simulink model "Boeing787_Yue"  (R2013a)
settings: Solver=ode23tb  SolverMode=SingleTasking  StartTime=0.0  StopTime=346  RelTol=1e-3
InitFcn:
  | load('SampleOutput.mat')
  | 
  | load('SampleFuelBurn.mat')
values from neighbouring files (symbols this model uses):
  FuelBurn = [0 0 0 0 0 0 0 0 0 0 0 0 ... (18249 elements, 1x18249)]    [Benchmark_data1.mat]
undefined symbols (not defined in the file or in its folder): ailerons, AirProp, B_737, elevator, HydProp, landing_gear, rudder, thrust_rev
libraries: PowerFlowLib x118, simulink x20
(part 25 of 26)

== system Boeing787_Yue/Electrical/Generation Unit Sync-Sync2/Generator/Stator Voltage ==
  Id : Inport
  Iq : Inport  Port=2
  Eq1 : Inport  Port=3
  Ed1 : Inport  Port=4
  Phi_1d : Inport  Port=5
  Phi_2q : Inport  Port=6
  w/ws : Inport  Port=7
  Temp : Inport  Port=8
  Gain : Gain  Gain=(Xq2 - Xls)/(Xq1 - Xls)
  Gain1 : Gain  Gain=(Xq1 - Xq2)/(Xq1 - Xls)
  Gain2 : Gain  Gain=(Xq2 - Xd2)
  Gain3 : Gain  Gain=(Xd2 - Xls)/(Xd1 - Xls)
  Gain4 : Gain  Gain=(Xd1 - Xd2)/(Xd1 - Xls)
  Gain5 : Gain  Gain=Rs
  Gain6 : Gain  Gain=Xd2
  Gain7 : Gain  Gain=Rs
  Gain8 : Gain  Gain=Xd2
  Product{,1..3,5} (5 alike) : Product  RndMeth=Zero
  Product4 : Product
  Sum : Sum
  Sum1 : Sum  Inputs=+-+
  Sum2 : Sum  Inputs=--+
  Sum3 : Sum  Inputs=-++
  Ed : Outport
  Eq : Outport  Port=2
  wires:
  Gain7/1 -> Sum2/2
  Product3/1 -> Sum2/1
  Sum2/1 -> Eq/1  "Vq"
  Sum3/1 -> Ed/1  "Vd"
  Product2/1 -> Sum3/3
  Product1/1 -> Sum3/2
  Gain8/1 -> Product3/1
  Gain6/1 -> Product2/2
  Id/1 -> Gain8/1, Gain5/1
  Product/1 -> Sum2/3
  w/ws/1 -> Product2/1, Product3/2, Product/2, Product1/2
  Sum1/1 -> Product1/1
  Sum/1 -> Product/1
  Gain1/1 -> Sum1/2
  Gain/1 -> Sum1/1
  Gain3/1 -> Sum/1
  Gain4/1 -> Sum/2
  Phi_1d/1 -> Gain4/1
  Eq1/1 -> Gain3/1
  Phi_2q/1 -> Gain1/1
  Ed1/1 -> Gain/1
  Gain2/1 -> Sum1/3
  Temp/1 -> Product5/1, Product4/2
  Gain5/1 -> Product4/1
  Product4/1 -> Sum3/1
  Product5/1 -> Gain7/1
  Iq/1 -> Gain2/1, Product5/2, Gain6/1

== system Boeing787_Yue/Electrical/Generation Unit Sync-Sync3/Generator/Dynamics ==
  Id : Inport
  Iq : Inport  Port=2
  Efd : Inport  Port=3
  Temp : Inport  Port=4
  Gain : Gain  Gain=Xd1 - Xls
  Gain1 : Gain  Gain=(Xd1 - Xd2)/(Xd1-Xls)^2
  Gain10 : Gain  Gain=Xq1 - Xls
  Gain11 : Gain  Gain=1/Tqo2
  Gain2 : Gain  Gain=Xd - Xd1
  Gain3 : Gain  Gain=1/Tdo1
  Gain4 : Gain  Gain=Xq1 - Xls
  Gain5 : Gain  Gain=(Xq1 - Xq2)/(Xq1 - Xls)^2
  Gain6 : Gain  Gain=Xq - Xq1
  Gain7 : Gain  Gain=1/Tqo1
  Gain8 : Gain  Gain=Xd1 - Xls
  Gain9 : Gain  Gain=1/Tdo2
  Integrator{,1..3} (4 alike) : Integrator
  Product{1..4} (4 alike) : Product
  Sum : Sum  Inputs=++-
  Sum1 : Sum  Inputs=+-
  Sum2 : Sum  Inputs=--+
  Sum3 : Sum  Inputs=+++
  Sum4 : Sum  Inputs=+-
  Sum5 : Sum  Inputs=-+
  Sum6 : Sum  Inputs=--+
  Sum7 : Sum  Inputs=---
  Eq1 : Outport
  Ed1 : Outport  Port=2
  Phi_1d : Outport  Port=3
  Phi_2q : Outport  Port=4
  wires:
  Efd/1 -> [Efd]
  Iq/1 -> [Iq]
  Id/1 -> [Id]
  Integrator3/1 -> Phi_2q/1, [Phi_2q]
  Sum7/1 -> Gain11/1
  [Ed1] -> Sum7/3
  [Phi_2q] -> Sum7/2
  Gain10/1 -> Sum7/1
  [Iq] -> Gain10/1
  Integrator2/1 -> Phi_1d/1, [Phi_1d]
  Sum6/1 -> Gain9/1
  [Eq1] -> Sum6/3
  [Phi_1d] -> Sum6/2
  Gain8/1 -> Sum6/1
  [Id] -> Gain8/1
  Sum5/1 -> Gain7/1
  Gain6/1 -> Sum5/2
  [Ed1] -> Sum5/1
  Sum4/1 -> Gain6/1
  Gain5/1 -> Sum4/2
  [Iq] -> Sum4/1
  Sum3/1 -> Gain5/1
  [Ed1] -> Sum3/3
  [Phi_2q] -> Sum3/2
  Gain4/1 -> Sum3/1
  [Iq] -> Gain4/1
  Integrator1/1 -> [Ed1], Ed1/1
  Sum2/1 -> Gain3/1
  [Efd] -> Sum2/3
  Gain2/1 -> Sum2/2
  [Eq1] -> Sum2/1
  Sum1/1 -> Gain2/1
  Gain1/1 -> Sum1/2
  [Id] -> Sum1/1
  Sum/1 -> Gain1/1
  [Eq1] -> Sum/3
  [Id] -> Gain/1
  Integrator/1 -> [Eq1], Eq1/1
  Gain/1 -> Sum/1
  [Phi_1d] -> Sum/2
  Temp/1 -> [R_temp_delta]
  [R_temp_delta] -> Product3/1
  Gain9/1 -> Product3/2
  Product3/1 -> Integrator2/1
  [R_temp_delta] -> Product1/1
  Gain11/1 -> Product1/2
  Product1/1 -> Integrator3/1
  [R_temp_delta] -> Product2/1
  Gain3/1 -> Product2/2
  Product2/1 -> Integrator/1
  [R_temp_delta] -> Product4/1
  Gain7/1 -> Product4/2
  Product4/1 -> Integrator1/1

== system Boeing787_Yue/Electrical/Generation Unit Sync-Sync3/Generator/Electromagnetic Torque Output Power ==
  note: Torque from Damper Windings
  note: Torque from Field Winding
  Id : Inport
  Iq : Inport  Port=2
  Eq1 : Inport  Port=3
  Ed1 : Inport  Port=4
  Phi_1d : Inport  Port=5
  Phi_2q : Inport  Port=6
  Gain : Gain  Gain=(Xd2 - Xls)/(Xd1 - Xls)
  Gain1 : Gain  Gain=(Xq2 - Xls)/(Xq1 - Xls)
  Gain2 : Gain  Gain=(Xd1 - Xd2)/(Xd1-Xls)
  Gain3 : Gain  Gain=(Xq1 - Xq2)/(Xq1-Xls)
  Gain4 : Gain  Gain=(Xq2 - Xd2)
  Product{,1..4} (5 alike) : Product  RndMeth=Zero
  Sum : Sum
  Sum1 : Sum  Inputs=+-+
  Sum2 : Sum
  TE : Outport
  wires:
  Sum2/1 -> TE/1
  Sum1/1 -> Sum2/2
  Sum/1 -> Sum2/1
  Gain1/1 -> Sum/2
  Gain/1 -> Sum/1
  Gain4/1 -> Sum1/3
  Gain2/1 -> Sum1/1
  Gain3/1 -> Sum1/2
  Product4/1 -> Gain4/1
  [Iq] -> Product4/2
  [Id] -> Product4/1
  Product3/1 -> Gain3/1
  [Phi_2q] -> Product3/2
  [Id] -> Product3/1
  Product2/1 -> Gain2/1
  [Phi_1d] -> Product2/2
  [Iq] -> Product2/1
  Product1/1 -> Gain1/1
  [Id] -> Product1/2
  [Ed1] -> Product1/1
  Product/1 -> Gain/1
  [Iq] -> Product/2
  [Eq1] -> Product/1
  Iq/1 -> [Iq]
  Phi_2q/1 -> [Phi_2q]
  Phi_1d/1 -> [Phi_1d]
  Ed1/1 -> [Ed1]
  Eq1/1 -> [Eq1]
  Id/1 -> [Id]

== system Boeing787_Yue/Electrical/Generation Unit Sync-Sync3/Generator/Generator Power Loss ==
  Ed : Inport
  Eq : Inport  Port=2
  Id : Inport  Port=3
  Iq : Inport  Port=4
  Te : Inport  Port=5
  w/ws : Inport  Port=6
  Bus Creator : BusCreator  Inputs=6
  Gain1 : Gain  Gain=SB
  Gain2 : Gain  Gain=SB
  Gain3 : Gain  Gain=SB
  Product : Product  RndMeth=Zero
  Product1 : Product  RndMeth=Zero
  Product2 : Product  RndMeth=Zero
  Sum1 : Sum  Inputs=-+
  Sum2 : Sum
  PE : Outport
  PM : Outport  Port=2
  PLOSS : Outport  Port=3
  m : Outport  Port=4
  wires:
  Gain3/1 -> PM/1
  Gain1/1 -> PE/1
  Gain2/1 -> PLOSS/1
  Bus Creator/1 -> m/1
  [nu] -> Bus Creator/6  "nu"
  [Te] -> Bus Creator/5  "Te"
  [Iq] -> Bus Creator/4  "Iq"
  [Eq] -> Bus Creator/3  "Vq"
  [Id] -> Bus Creator/2  "Id"
  [Ed] -> Bus Creator/1  "Vd"
  Sum1/1 -> Gain2/1
  Product2/1 -> Gain3/1, Sum1/2
  Sum2/1 -> Gain1/1, Sum1/1
  Product1/1 -> Sum2/2
  Product/1 -> Sum2/1
  [nu] -> Product2/2
  [Te] -> Product2/1
  [Iq] -> Product1/2
  [Eq] -> Product1/1
  [Id] -> Product/2
  [Ed] -> Product/1
  w/ws/1 -> [nu]
  Te/1 -> [Te]
  Iq/1 -> [Iq]
  Id/1 -> [Id]
  Eq/1 -> [Eq]
  Ed/1 -> [Ed]

== system Boeing787_Yue/Electrical/Generation Unit Sync-Sync3/Generator/Stator Voltage ==
  Id : Inport
  Iq : Inport  Port=2
  Eq1 : Inport  Port=3
  Ed1 : Inport  Port=4
  Phi_1d : Inport  Port=5
  Phi_2q : Inport  Port=6
  w/ws : Inport  Port=7
  Temp : Inport  Port=8
  Gain : Gain  Gain=(Xq2 - Xls)/(Xq1 - Xls)
  Gain1 : Gain  Gain=(Xq1 - Xq2)/(Xq1 - Xls)
  Gain2 : Gain  Gain=(Xq2 - Xd2)
  Gain3 : Gain  Gain=(Xd2 - Xls)/(Xd1 - Xls)
  Gain4 : Gain  Gain=(Xd1 - Xd2)/(Xd1 - Xls)
  Gain5 : Gain  Gain=Rs
  Gain6 : Gain  Gain=Xd2
  Gain7 : Gain  Gain=Rs
  Gain8 : Gain  Gain=Xd2
  Product{,1..3,5} (5 alike) : Product  RndMeth=Zero
  Product4 : Product
  Sum : Sum
  Sum1 : Sum  Inputs=+-+
  Sum2 : Sum  Inputs=--+
  Sum3 : Sum  Inputs=-++
  Ed : Outport
  Eq : Outport  Port=2
  wires:
  Gain7/1 -> Sum2/2
  Product3/1 -> Sum2/1
  Sum2/1 -> Eq/1  "Vq"
  Sum3/1 -> Ed/1  "Vd"
  Product2/1 -> Sum3/3
  Product1/1 -> Sum3/2
  Gain8/1 -> Product3/1
  Gain6/1 -> Product2/2
  Id/1 -> Gain8/1, Gain5/1
  Product/1 -> Sum2/3
  w/ws/1 -> Product2/1, Product3/2, Product/2, Product1/2
  Sum1/1 -> Product1/1
  Sum/1 -> Product/1
  Gain1/1 -> Sum1/2
  Gain/1 -> Sum1/1
  Gain3/1 -> Sum/1
  Gain4/1 -> Sum/2
  Phi_1d/1 -> Gain4/1
  Eq1/1 -> Gain3/1
  Phi_2q/1 -> Gain1/1
  Ed1/1 -> Gain/1
  Gain2/1 -> Sum1/3
  Temp/1 -> Product5/1, Product4/2
  Gain5/1 -> Product4/1
  Product4/1 -> Sum3/1
  Product5/1 -> Gain7/1
  Iq/1 -> Gain2/1, Product5/2, Gain6/1

== system Boeing787_Yue/Electrical/Generation Unit Sync-Sync4/Generator/Dynamics ==
  Id : Inport
  Iq : Inport  Port=2
  Efd : Inport  Port=3
  Temp : Inport  Port=4
  Gain : Gain  Gain=Xd1 - Xls
  Gain1 : Gain  Gain=(Xd1 - Xd2)/(Xd1-Xls)^2
  Gain10 : Gain  Gain=Xq1 - Xls
  Gain11 : Gain  Gain=1/Tqo2
  Gain2 : Gain  Gain=Xd - Xd1
  Gain3 : Gain  Gain=1/Tdo1
  Gain4 : Gain  Gain=Xq1 - Xls
  Gain5 : Gain  Gain=(Xq1 - Xq2)/(Xq1 - Xls)^2
  Gain6 : Gain  Gain=Xq - Xq1
  Gain7 : Gain  Gain=1/Tqo1
  Gain8 : Gain  Gain=Xd1 - Xls
  Gain9 : Gain  Gain=1/Tdo2
  Integrator{,1..3} (4 alike) : Integrator
  Product{1..4} (4 alike) : Product
  Sum : Sum  Inputs=++-
  Sum1 : Sum  Inputs=+-
  Sum2 : Sum  Inputs=--+
  Sum3 : Sum  Inputs=+++
  Sum4 : Sum  Inputs=+-
  Sum5 : Sum  Inputs=-+
  Sum6 : Sum  Inputs=--+
  Sum7 : Sum  Inputs=---
  Eq1 : Outport
  Ed1 : Outport  Port=2
  Phi_1d : Outport  Port=3
  Phi_2q : Outport  Port=4
  wires:
  Efd/1 -> [Efd]
  Iq/1 -> [Iq]
  Id/1 -> [Id]
  Integrator3/1 -> Phi_2q/1, [Phi_2q]
  Sum7/1 -> Gain11/1
  [Ed1] -> Sum7/3
  [Phi_2q] -> Sum7/2
  Gain10/1 -> Sum7/1
  [Iq] -> Gain10/1
  Integrator2/1 -> Phi_1d/1, [Phi_1d]
  Sum6/1 -> Gain9/1
  [Eq1] -> Sum6/3
  [Phi_1d] -> Sum6/2
  Gain8/1 -> Sum6/1
  [Id] -> Gain8/1
  Sum5/1 -> Gain7/1
  Gain6/1 -> Sum5/2
  [Ed1] -> Sum5/1
  Sum4/1 -> Gain6/1
  Gain5/1 -> Sum4/2
  [Iq] -> Sum4/1
  Sum3/1 -> Gain5/1
  [Ed1] -> Sum3/3
  [Phi_2q] -> Sum3/2
  Gain4/1 -> Sum3/1
  [Iq] -> Gain4/1
  Integrator1/1 -> [Ed1], Ed1/1
  Sum2/1 -> Gain3/1
  [Efd] -> Sum2/3
  Gain2/1 -> Sum2/2
  [Eq1] -> Sum2/1
  Sum1/1 -> Gain2/1
  Gain1/1 -> Sum1/2
  [Id] -> Sum1/1
  Sum/1 -> Gain1/1
  [Eq1] -> Sum/3
  [Id] -> Gain/1
  Integrator/1 -> [Eq1], Eq1/1
  Gain/1 -> Sum/1
  [Phi_1d] -> Sum/2
  Temp/1 -> [R_temp_delta]
  [R_temp_delta] -> Product3/1
  Gain9/1 -> Product3/2
  Product3/1 -> Integrator2/1
  [R_temp_delta] -> Product1/1
  Gain11/1 -> Product1/2
  Product1/1 -> Integrator3/1
  [R_temp_delta] -> Product2/1
  Gain3/1 -> Product2/2
  Product2/1 -> Integrator/1
  [R_temp_delta] -> Product4/1
  Gain7/1 -> Product4/2
  Product4/1 -> Integrator1/1

== system Boeing787_Yue/Electrical/Generation Unit Sync-Sync4/Generator/Electromagnetic Torque Output Power ==
  note: Torque from Damper Windings
  note: Torque from Field Winding
  Id : Inport
  Iq : Inport  Port=2
  Eq1 : Inport  Port=3
  Ed1 : Inport  Port=4
  Phi_1d : Inport  Port=5
  Phi_2q : Inport  Port=6
  Gain : Gain  Gain=(Xd2 - Xls)/(Xd1 - Xls)
  Gain1 : Gain  Gain=(Xq2 - Xls)/(Xq1 - Xls)
  Gain2 : Gain  Gain=(Xd1 - Xd2)/(Xd1-Xls)
  Gain3 : Gain  Gain=(Xq1 - Xq2)/(Xq1-Xls)
  Gain4 : Gain  Gain=(Xq2 - Xd2)
  Product{,1..4} (5 alike) : Product  RndMeth=Zero
  Sum : Sum
  Sum1 : Sum  Inputs=+-+
  Sum2 : Sum
  TE : Outport
  wires:
  Sum2/1 -> TE/1
  Sum1/1 -> Sum2/2
  Sum/1 -> Sum2/1
  Gain1/1 -> Sum/2
  Gain/1 -> Sum/1
  Gain4/1 -> Sum1/3
  Gain2/1 -> Sum1/1
  Gain3/1 -> Sum1/2
  Product4/1 -> Gain4/1
  [Iq] -> Product4/2
  [Id] -> Product4/1
  Product3/1 -> Gain3/1
  [Phi_2q] -> Product3/2
  [Id] -> Product3/1
  Product2/1 -> Gain2/1
  [Phi_1d] -> Product2/2
  [Iq] -> Product2/1
  Product1/1 -> Gain1/1
  [Id] -> Product1/2
  [Ed1] -> Product1/1
  Product/1 -> Gain/1
  [Iq] -> Product/2
  [Eq1] -> Product/1
  Iq/1 -> [Iq]
  Phi_2q/1 -> [Phi_2q]
  Phi_1d/1 -> [Phi_1d]
  Ed1/1 -> [Ed1]
  Eq1/1 -> [Eq1]
  Id/1 -> [Id]

== system Boeing787_Yue/Electrical/Generation Unit Sync-Sync4/Generator/Generator Power Loss ==
  Ed : Inport
  Eq : Inport  Port=2
  Id : Inport  Port=3
  Iq : Inport  Port=4
  Te : Inport  Port=5
  w/ws : Inport  Port=6
  Bus Creator : BusCreator  Inputs=6
  Gain1 : Gain  Gain=SB
  Gain2 : Gain  Gain=SB
  Gain3 : Gain  Gain=SB
  Product : Product  RndMeth=Zero
  Product1 : Product  RndMeth=Zero
  Product2 : Product  RndMeth=Zero
  Sum1 : Sum  Inputs=-+
  Sum2 : Sum
  PE : Outport
  PM : Outport  Port=2
  PLOSS : Outport  Port=3
  m : Outport  Port=4
  wires:
  Gain3/1 -> PM/1
  Gain1/1 -> PE/1
  Gain2/1 -> PLOSS/1
  Bus Creator/1 -> m/1
  [nu] -> Bus Creator/6  "nu"
  [Te] -> Bus Creator/5  "Te"
  [Iq] -> Bus Creator/4  "Iq"
  [Eq] -> Bus Creator/3  "Vq"
  [Id] -> Bus Creator/2  "Id"
  [Ed] -> Bus Creator/1  "Vd"
  Sum1/1 -> Gain2/1
  Product2/1 -> Gain3/1, Sum1/2
  Sum2/1 -> Gain1/1, Sum1/1
  Product1/1 -> Sum2/2
  Product/1 -> Sum2/1
  [nu] -> Product2/2
  [Te] -> Product2/1
  [Iq] -> Product1/2
  [Eq] -> Product1/1
  [Id] -> Product/2
  [Ed] -> Product/1
  w/ws/1 -> [nu]
  Te/1 -> [Te]
  Iq/1 -> [Iq]
  Id/1 -> [Id]
  Eq/1 -> [Eq]
  Ed/1 -> [Ed]

== system Boeing787_Yue/Electrical/Generation Unit Sync-Sync4/Generator/Stator Voltage ==
  Id : Inport
  Iq : Inport  Port=2
  Eq1 : Inport  Port=3
  Ed1 : Inport  Port=4
  Phi_1d : Inport  Port=5
  Phi_2q : Inport  Port=6
  w/ws : Inport  Port=7
  Temp : Inport  Port=8
  Gain : Gain  Gain=(Xq2 - Xls)/(Xq1 - Xls)
  Gain1 : Gain  Gain=(Xq1 - Xq2)/(Xq1 - Xls)
  Gain2 : Gain  Gain=(Xq2 - Xd2)
  Gain3 : Gain  Gain=(Xd2 - Xls)/(Xd1 - Xls)
  Gain4 : Gain  Gain=(Xd1 - Xd2)/(Xd1 - Xls)
  Gain5 : Gain  Gain=Rs
  Gain6 : Gain  Gain=Xd2
  Gain7 : Gain  Gain=Rs
  Gain8 : Gain  Gain=Xd2
  Product{,1..3,5} (5 alike) : Product  RndMeth=Zero
  Product4 : Product
  Sum : Sum
  Sum1 : Sum  Inputs=+-+
  Sum2 : Sum  Inputs=--+
  Sum3 : Sum  Inputs=-++
  Ed : Outport
  Eq : Outport  Port=2
  wires:
  Gain7/1 -> Sum2/2
  Product3/1 -> Sum2/1
  Sum2/1 -> Eq/1  "Vq"
  Sum3/1 -> Ed/1  "Vd"
  Product2/1 -> Sum3/3
  Product1/1 -> Sum3/2
  Gain8/1 -> Product3/1
  Gain6/1 -> Product2/2
  Id/1 -> Gain8/1, Gain5/1
  Product/1 -> Sum2/3
  w/ws/1 -> Product2/1, Product3/2, Product/2, Product1/2
  Sum1/1 -> Product1/1
  Sum/1 -> Product/1
  Gain1/1 -> Sum1/2
  Gain/1 -> Sum1/1
  Gain3/1 -> Sum/1
  Gain4/1 -> Sum/2
  Phi_1d/1 -> Gain4/1
  Eq1/1 -> Gain3/1
  Phi_2q/1 -> Gain1/1
  Ed1/1 -> Gain/1
  Gain2/1 -> Sum1/3
  Temp/1 -> Product5/1, Product4/2
  Gain5/1 -> Product4/1
  Product4/1 -> Sum3/1
  Product5/1 -> Gain7/1
  Iq/1 -> Gain2/1, Product5/2, Gain6/1

== system Boeing787_Yue/Electrical/Generation Unit Sync-Sync5/Generator/Dynamics ==
  Id : Inport
  Iq : Inport  Port=2
  Efd : Inport  Port=3
  Temp : Inport  Port=4
  Gain : Gain  Gain=Xd1 - Xls
  Gain1 : Gain  Gain=(Xd1 - Xd2)/(Xd1-Xls)^2
  Gain10 : Gain  Gain=Xq1 - Xls
  Gain11 : Gain  Gain=1/Tqo2
  Gain2 : Gain  Gain=Xd - Xd1
  Gain3 : Gain  Gain=1/Tdo1
  Gain4 : Gain  Gain=Xq1 - Xls
  Gain5 : Gain  Gain=(Xq1 - Xq2)/(Xq1 - Xls)^2
  Gain6 : Gain  Gain=Xq - Xq1
  Gain7 : Gain  Gain=1/Tqo1
  Gain8 : Gain  Gain=Xd1 - Xls
  Gain9 : Gain  Gain=1/Tdo2
  Integrator{,1..3} (4 alike) : Integrator
  Product{1..4} (4 alike) : Product
  Sum : Sum  Inputs=++-
  Sum1 : Sum  Inputs=+-
  Sum2 : Sum  Inputs=--+
  Sum3 : Sum  Inputs=+++
  Sum4 : Sum  Inputs=+-
  Sum5 : Sum  Inputs=-+
  Sum6 : Sum  Inputs=--+
  Sum7 : Sum  Inputs=---
  Eq1 : Outport
  Ed1 : Outport  Port=2
  Phi_1d : Outport  Port=3
  Phi_2q : Outport  Port=4
  wires:
  Efd/1 -> [Efd]
  Iq/1 -> [Iq]
  Id/1 -> [Id]
  Integrator3/1 -> Phi_2q/1, [Phi_2q]
  Sum7/1 -> Gain11/1
  [Ed1] -> Sum7/3
  [Phi_2q] -> Sum7/2
  Gain10/1 -> Sum7/1
  [Iq] -> Gain10/1
  Integrator2/1 -> Phi_1d/1, [Phi_1d]
  Sum6/1 -> Gain9/1
  [Eq1] -> Sum6/3
  [Phi_1d] -> Sum6/2
  Gain8/1 -> Sum6/1
  [Id] -> Gain8/1
  Sum5/1 -> Gain7/1
  Gain6/1 -> Sum5/2
  [Ed1] -> Sum5/1
  Sum4/1 -> Gain6/1
  Gain5/1 -> Sum4/2
  [Iq] -> Sum4/1
  Sum3/1 -> Gain5/1
  [Ed1] -> Sum3/3
  [Phi_2q] -> Sum3/2
  Gain4/1 -> Sum3/1
  [Iq] -> Gain4/1
  Integrator1/1 -> [Ed1], Ed1/1
  Sum2/1 -> Gain3/1
  [Efd] -> Sum2/3
  Gain2/1 -> Sum2/2
  [Eq1] -> Sum2/1
  Sum1/1 -> Gain2/1
  Gain1/1 -> Sum1/2
  [Id] -> Sum1/1
  Sum/1 -> Gain1/1
  [Eq1] -> Sum/3
  [Id] -> Gain/1
  Integrator/1 -> [Eq1], Eq1/1
  Gain/1 -> Sum/1
  [Phi_1d] -> Sum/2
  Temp/1 -> [R_temp_delta]
  [R_temp_delta] -> Product3/1
  Gain9/1 -> Product3/2
  Product3/1 -> Integrator2/1
  [R_temp_delta] -> Product1/1
  Gain11/1 -> Product1/2
  Product1/1 -> Integrator3/1
  [R_temp_delta] -> Product2/1
  Gain3/1 -> Product2/2
  Product2/1 -> Integrator/1
  [R_temp_delta] -> Product4/1
  Gain7/1 -> Product4/2
  Product4/1 -> Integrator1/1

== system Boeing787_Yue/Electrical/Generation Unit Sync-Sync5/Generator/Electromagnetic Torque Output Power ==
  note: Torque from Damper Windings
  note: Torque from Field Winding
  Id : Inport
  Iq : Inport  Port=2
  Eq1 : Inport  Port=3
  Ed1 : Inport  Port=4
  Phi_1d : Inport  Port=5
  Phi_2q : Inport  Port=6
  Gain : Gain  Gain=(Xd2 - Xls)/(Xd1 - Xls)
  Gain1 : Gain  Gain=(Xq2 - Xls)/(Xq1 - Xls)
  Gain2 : Gain  Gain=(Xd1 - Xd2)/(Xd1-Xls)
  Gain3 : Gain  Gain=(Xq1 - Xq2)/(Xq1-Xls)
  Gain4 : Gain  Gain=(Xq2 - Xd2)
  Product{,1..4} (5 alike) : Product  RndMeth=Zero
  Sum : Sum
  Sum1 : Sum  Inputs=+-+
  Sum2 : Sum
  TE : Outport
  wires:
  Sum2/1 -> TE/1
  Sum1/1 -> Sum2/2
  Sum/1 -> Sum2/1
  Gain1/1 -> Sum/2
  Gain/1 -> Sum/1
  Gain4/1 -> Sum1/3
  Gain2/1 -> Sum1/1
  Gain3/1 -> Sum1/2
  Product4/1 -> Gain4/1
  [Iq] -> Product4/2
  [Id] -> Product4/1
  Product3/1 -> Gain3/1
  [Phi_2q] -> Product3/2
  [Id] -> Product3/1
  Product2/1 -> Gain2/1
  [Phi_1d] -> Product2/2
  [Iq] -> Product2/1
  Product1/1 -> Gain1/1
  [Id] -> Product1/2
  [Ed1] -> Product1/1
  Product/1 -> Gain/1
  [Iq] -> Product/2
  [Eq1] -> Product/1
  Iq/1 -> [Iq]
  Phi_2q/1 -> [Phi_2q]
  Phi_1d/1 -> [Phi_1d]
  Ed1/1 -> [Ed1]
  Eq1/1 -> [Eq1]
  Id/1 -> [Id]

== system Boeing787_Yue/Electrical/Generation Unit Sync-Sync5/Generator/Generator Power Loss ==
  Ed : Inport
  Eq : Inport  Port=2
  Id : Inport  Port=3
  Iq : Inport  Port=4
  Te : Inport  Port=5
  w/ws : Inport  Port=6
  Bus Creator : BusCreator  Inputs=6
  Gain1 : Gain  Gain=SB
  Gain2 : Gain  Gain=SB
  Gain3 : Gain  Gain=SB
  Product : Product  RndMeth=Zero
  Product1 : Product  RndMeth=Zero
  Product2 : Product  RndMeth=Zero
  Sum1 : Sum  Inputs=-+
  Sum2 : Sum
  PE : Outport
  PM : Outport  Port=2
  PLOSS : Outport  Port=3
  m : Outport  Port=4
  wires:
  Gain3/1 -> PM/1
  Gain1/1 -> PE/1
  Gain2/1 -> PLOSS/1
  Bus Creator/1 -> m/1
  [nu] -> Bus Creator/6  "nu"
  [Te] -> Bus Creator/5  "Te"
  [Iq] -> Bus Creator/4  "Iq"
  [Eq] -> Bus Creator/3  "Vq"
  [Id] -> Bus Creator/2  "Id"
  [Ed] -> Bus Creator/1  "Vd"
  Sum1/1 -> Gain2/1
  Product2/1 -> Gain3/1, Sum1/2
  Sum2/1 -> Gain1/1, Sum1/1
  Product1/1 -> Sum2/2
  Product/1 -> Sum2/1
  [nu] -> Product2/2
  [Te] -> Product2/1
  [Iq] -> Product1/2
  [Eq] -> Product1/1
  [Id] -> Product/2
  [Ed] -> Product/1
  w/ws/1 -> [nu]
  Te/1 -> [Te]
  Iq/1 -> [Iq]
  Id/1 -> [Id]
  Eq/1 -> [Eq]
  Ed/1 -> [Ed]

== system Boeing787_Yue/Electrical/Generation Unit Sync-Sync5/Generator/Stator Voltage ==
  Id : Inport
  Iq : Inport  Port=2
  Eq1 : Inport  Port=3
  Ed1 : Inport  Port=4
  Phi_1d : Inport  Port=5
  Phi_2q : Inport  Port=6
  w/ws : Inport  Port=7
  Temp : Inport  Port=8
  Gain : Gain  Gain=(Xq2 - Xls)/(Xq1 - Xls)
  Gain1 : Gain  Gain=(Xq1 - Xq2)/(Xq1 - Xls)
  Gain2 : Gain  Gain=(Xq2 - Xd2)
  Gain3 : Gain  Gain=(Xd2 - Xls)/(Xd1 - Xls)
  Gain4 : Gain  Gain=(Xd1 - Xd2)/(Xd1 - Xls)
  Gain5 : Gain  Gain=Rs
  Gain6 : Gain  Gain=Xd2
  Gain7 : Gain  Gain=Rs
  Gain8 : Gain  Gain=Xd2
  Product{,1..3,5} (5 alike) : Product  RndMeth=Zero
  Product4 : Product
  Sum : Sum
  Sum1 : Sum  Inputs=+-+
  Sum2 : Sum  Inputs=--+
  Sum3 : Sum  Inputs=-++
  Ed : Outport
  Eq : Outport  Port=2
  wires:
  Gain7/1 -> Sum2/2
  Product3/1 -> Sum2/1
  Sum2/1 -> Eq/1  "Vq"
  Sum3/1 -> Ed/1  "Vd"
  Product2/1 -> Sum3/3
  Product1/1 -> Sum3/2
  Gain8/1 -> Product3/1
  Gain6/1 -> Product2/2
  Id/1 -> Gain8/1, Gain5/1
  Product/1 -> Sum2/3
  w/ws/1 -> Product2/1, Product3/2, Product/2, Product1/2
  Sum1/1 -> Product1/1
  Sum/1 -> Product/1
  Gain1/1 -> Sum1/2
  Gain/1 -> Sum1/1
  Gain3/1 -> Sum/1
  Gain4/1 -> Sum/2
  Phi_1d/1 -> Gain4/1
  Eq1/1 -> Gain3/1
  Phi_2q/1 -> Gain1/1
  Ed1/1 -> Gain/1
  Gain2/1 -> Sum1/3
  Temp/1 -> Product5/1, Product4/2
  Gain5/1 -> Product4/1
  Product4/1 -> Sum3/1
  Product5/1 -> Gain7/1
  Iq/1 -> Gain2/1, Product5/2, Gain6/1

== system Boeing787_Yue/Electrical/Generation Unit Sync-Sync6/Generator/Dynamics ==
  Id : Inport
  Iq : Inport  Port=2
  Efd : Inport  Port=3
  Temp : Inport  Port=4
  Gain : Gain  Gain=Xd1 - Xls
  Gain1 : Gain  Gain=(Xd1 - Xd2)/(Xd1-Xls)^2
  Gain10 : Gain  Gain=Xq1 - Xls
  Gain11 : Gain  Gain=1/Tqo2
  Gain2 : Gain  Gain=Xd - Xd1
  Gain3 : Gain  Gain=1/Tdo1
  Gain4 : Gain  Gain=Xq1 - Xls
  Gain5 : Gain  Gain=(Xq1 - Xq2)/(Xq1 - Xls)^2
  Gain6 : Gain  Gain=Xq - Xq1
  Gain7 : Gain  Gain=1/Tqo1
  Gain8 : Gain  Gain=Xd1 - Xls
  Gain9 : Gain  Gain=1/Tdo2
  Integrator{,1..3} (4 alike) : Integrator
  Product{1..4} (4 alike) : Product
  Sum : Sum  Inputs=++-
  Sum1 : Sum  Inputs=+-
  Sum2 : Sum  Inputs=--+
  Sum3 : Sum  Inputs=+++
  Sum4 : Sum  Inputs=+-
  Sum5 : Sum  Inputs=-+
  Sum6 : Sum  Inputs=--+
  Sum7 : Sum  Inputs=---
  Eq1 : Outport
  Ed1 : Outport  Port=2
  Phi_1d : Outport  Port=3
  Phi_2q : Outport  Port=4
  wires:
  Product4/1 -> Integrator1/1
  Gain7/1 -> Product4/2
  [R_temp_delta] -> Product4/1
  Product2/1 -> Integrator/1
  Gain3/1 -> Product2/2
  [R_temp_delta] -> Product2/1
  Product1/1 -> Integrator3/1
  Gain11/1 -> Product1/2
  [R_temp_delta] -> Product1/1
  Product3/1 -> Integrator2/1
  Gain9/1 -> Product3/2
  [R_temp_delta] -> Product3/1
  Temp/1 -> [R_temp_delta]
  [Phi_1d] -> Sum/2
  Gain/1 -> Sum/1
  Integrator/1 -> Eq1/1, [Eq1]
  [Id] -> Gain/1
  [Eq1] -> Sum/3
  Sum/1 -> Gain1/1
  [Id] -> Sum1/1
  Gain1/1 -> Sum1/2
  Sum1/1 -> Gain2/1
  [Eq1] -> Sum2/1
  Gain2/1 -> Sum2/2
  [Efd] -> Sum2/3
  Sum2/1 -> Gain3/1
  Integrator1/1 -> Ed1/1, [Ed1]
  [Iq] -> Gain4/1
  Gain4/1 -> Sum3/1
  [Phi_2q] -> Sum3/2
  [Ed1] -> Sum3/3
  Sum3/1 -> Gain5/1
  [Iq] -> Sum4/1
  Gain5/1 -> Sum4/2
  Sum4/1 -> Gain6/1
  [Ed1] -> Sum5/1
  Gain6/1 -> Sum5/2
  Sum5/1 -> Gain7/1
  [Id] -> Gain8/1
  Gain8/1 -> Sum6/1
  [Phi_1d] -> Sum6/2
  [Eq1] -> Sum6/3
  Sum6/1 -> Gain9/1
  Integrator2/1 -> [Phi_1d], Phi_1d/1
  [Iq] -> Gain10/1
  Gain10/1 -> Sum7/1
  [Phi_2q] -> Sum7/2
  [Ed1] -> Sum7/3
  Sum7/1 -> Gain11/1
  Integrator3/1 -> [Phi_2q], Phi_2q/1
  Id/1 -> [Id]
  Iq/1 -> [Iq]
  Efd/1 -> [Efd]

== system Boeing787_Yue/Electrical/Generation Unit Sync-Sync6/Generator/Electromagnetic Torque Output Power ==
  note: Torque from Field Winding
  note: Torque from Damper Windings
  Id : Inport
  Iq : Inport  Port=2
  Eq1 : Inport  Port=3
  Ed1 : Inport  Port=4
  Phi_1d : Inport  Port=5
  Phi_2q : Inport  Port=6
  Gain : Gain  Gain=(Xd2 - Xls)/(Xd1 - Xls)
  Gain1 : Gain  Gain=(Xq2 - Xls)/(Xq1 - Xls)
  Gain2 : Gain  Gain=(Xd1 - Xd2)/(Xd1-Xls)
  Gain3 : Gain  Gain=(Xq1 - Xq2)/(Xq1-Xls)
  Gain4 : Gain  Gain=(Xq2 - Xd2)
  Product{,1..4} (5 alike) : Product  RndMeth=Zero
  Sum : Sum
  Sum1 : Sum  Inputs=+-+
  Sum2 : Sum
  TE : Outport
  wires:
  Id/1 -> [Id]
  Eq1/1 -> [Eq1]
  Ed1/1 -> [Ed1]
  Phi_1d/1 -> [Phi_1d]
  Phi_2q/1 -> [Phi_2q]
  Iq/1 -> [Iq]
  [Eq1] -> Product/1
  [Iq] -> Product/2
  Product/1 -> Gain/1
  [Ed1] -> Product1/1
  [Id] -> Product1/2
  Product1/1 -> Gain1/1
  [Iq] -> Product2/1
  [Phi_1d] -> Product2/2
  Product2/1 -> Gain2/1
  [Id] -> Product3/1
  [Phi_2q] -> Product3/2
  Product3/1 -> Gain3/1
  [Id] -> Product4/1
  [Iq] -> Product4/2
  Product4/1 -> Gain4/1
  Gain3/1 -> Sum1/2
  Gain2/1 -> Sum1/1
  Gain4/1 -> Sum1/3
  Gain/1 -> Sum/1
  Gain1/1 -> Sum/2
  Sum/1 -> Sum2/1
  Sum1/1 -> Sum2/2
  Sum2/1 -> TE/1

== system Boeing787_Yue/Electrical/Generation Unit Sync-Sync6/Generator/Generator Power Loss ==
  Ed : Inport
  Eq : Inport  Port=2
  Id : Inport  Port=3
  Iq : Inport  Port=4
  Te : Inport  Port=5
  w/ws : Inport  Port=6
  Bus Creator : BusCreator  Inputs=6
  Gain1 : Gain  Gain=SB
  Gain2 : Gain  Gain=SB
  Gain3 : Gain  Gain=SB
  Product : Product  RndMeth=Zero
  Product1 : Product  RndMeth=Zero
  Product2 : Product  RndMeth=Zero
  Sum1 : Sum  Inputs=-+
  Sum2 : Sum
  PE : Outport
  PM : Outport  Port=2
  PLOSS : Outport  Port=3
  m : Outport  Port=4
  wires:
  Ed/1 -> [Ed]
  Eq/1 -> [Eq]
  Id/1 -> [Id]
  Iq/1 -> [Iq]
  Te/1 -> [Te]
  w/ws/1 -> [nu]
  [Ed] -> Product/1
  [Id] -> Product/2
  [Eq] -> Product1/1
  [Iq] -> Product1/2
  [Te] -> Product2/1
  [nu] -> Product2/2
  Product/1 -> Sum2/1
  Product1/1 -> Sum2/2
  Sum2/1 -> Sum1/1, Gain1/1
  Product2/1 -> Sum1/2, Gain3/1
  Sum1/1 -> Gain2/1
  [Ed] -> Bus Creator/1  "Vd"
  [Id] -> Bus Creator/2  "Id"
  [Eq] -> Bus Creator/3  "Vq"
  [Iq] -> Bus Creator/4  "Iq"
  [Te] -> Bus Creator/5  "Te"
  [nu] -> Bus Creator/6  "nu"
  Bus Creator/1 -> m/1
  Gain2/1 -> PLOSS/1
  Gain1/1 -> PE/1
  Gain3/1 -> PM/1

== system Boeing787_Yue/Electrical/Generation Unit Sync-Sync6/Generator/Stator Voltage ==
  Id : Inport
  Iq : Inport  Port=2
  Eq1 : Inport  Port=3
  Ed1 : Inport  Port=4
  Phi_1d : Inport  Port=5
  Phi_2q : Inport  Port=6
  w/ws : Inport  Port=7
  Temp : Inport  Port=8
  Gain : Gain  Gain=(Xq2 - Xls)/(Xq1 - Xls)
  Gain1 : Gain  Gain=(Xq1 - Xq2)/(Xq1 - Xls)
  Gain2 : Gain  Gain=(Xq2 - Xd2)
  Gain3 : Gain  Gain=(Xd2 - Xls)/(Xd1 - Xls)
  Gain4 : Gain  Gain=(Xd1 - Xd2)/(Xd1 - Xls)
  Gain5 : Gain  Gain=Rs
  Gain6 : Gain  Gain=Xd2
  Gain7 : Gain  Gain=Rs
  Gain8 : Gain  Gain=Xd2
  Product{,1..3,5} (5 alike) : Product  RndMeth=Zero
  Product4 : Product
  Sum : Sum
  Sum1 : Sum  Inputs=+-+
  Sum2 : Sum  Inputs=--+
  Sum3 : Sum  Inputs=-++
  Ed : Outport
  Eq : Outport  Port=2
  wires:
  Iq/1 -> Gain6/1, Product5/2, Gain2/1
  Product5/1 -> Gain7/1
  Product4/1 -> Sum3/1
  Gain5/1 -> Product4/1
  Temp/1 -> Product4/2, Product5/1
  Gain2/1 -> Sum1/3
  Ed1/1 -> Gain/1
  Phi_2q/1 -> Gain1/1
  Eq1/1 -> Gain3/1
  Phi_1d/1 -> Gain4/1
  Gain4/1 -> Sum/2
  Gain3/1 -> Sum/1
  Gain/1 -> Sum1/1
  Gain1/1 -> Sum1/2
  Sum/1 -> Product/1
  Sum1/1 -> Product1/1
  w/ws/1 -> Product1/2, Product/2, Product3/2, Product2/1
  Product/1 -> Sum2/3
  Id/1 -> Gain5/1, Gain8/1
  Gain6/1 -> Product2/2
  Gain8/1 -> Product3/1
  Product1/1 -> Sum3/2
  Product2/1 -> Sum3/3
  Sum3/1 -> Ed/1  "Vd"
  Sum2/1 -> Eq/1  "Vq"
  Product3/1 -> Sum2/1
  Gain7/1 -> Sum2/2

== system Boeing787_Yue/Hydraulic/Center Hydraulic System/DC Speed Servo/DC Machine ==
  note: Armature Current ia
  note: Field Current If
  Vf : Inport
  Va : Inport  Port=2
  Tload : Inport  Port=3
  Gain : Gain  Gain=Rfsh
  Gain1 : Gain  Gain=1/Lfsh
  Gain2 : Gain  Gain=Ra
  Gain3 : Gain  Gain=1/La
  Gain4 : Gain  Gain=1/J
  Gain7 : Gain  Gain=Lmsh
  Gain8 : Gain  Gain=Ra
  Gain9 : Gain  Gain=Rfsh
  Integrator : Integrator
  Integrator1 : Integrator
  Integrator2 : Integrator  InitialCondition=10  LimitOutput=on  LowerSaturationLimit=1
  Integrator3 : Integrator  ZeroCross=off
  Math Function1 : Math  Operator=square  SaturateOnIntegerOverflow=on
  Math Function2 : Math  Operator=square  SaturateOnIntegerOverflow=on
  Product{,1..4} (5 alike) : Product  RndMeth=Zero
  Sum : Sum  Inputs=|+-
  Sum1 : Sum  Inputs=-+-
  Sum2 : Sum  Inputs=+-
  Sum4 : Sum  Inputs=|++
  Sum5 : Sum  Inputs=|++
  Terminator : Terminator
  Terminator1 : Terminator
  If : Outport
  Ia : Outport  Port=2
  Pe : Outport  Port=3
  Pm : Outport  Port=4
  Plosses : Outport  Port=5
  Te : Outport  Port=6
  Speed : Outport  Port=7
  theta : Outport  Port=8
  wires:
  Integrator3/1 -> Terminator/1, theta/1
  Gain/1 -> Sum/2
  Sum/1 -> Gain1/1
  Integrator/1 -> Gain/1, [field_ct], If/1
  Sum1/1 -> Gain3/1
  Gain3/1 -> Integrator1/1
  Integrator1/1 -> Gain2/1, [arm_ct], Ia/1
  Product1/1 -> Sum2/1, Te/1
  Sum2/1 -> Gain4/1
  Gain4/1 -> Integrator2/1
  Gain1/1 -> Integrator/1
  Product/1 -> Sum1/1
  Gain2/1 -> Sum1/3
  [lambdaf] -> Product1/1
  [arm_ct] -> Product1/2
  [load_torque] -> Sum2/2
  [speed] -> Product/2
  [lambdaf] -> Product/1
  [field_ct] -> Gain7/1
  Gain7/1 -> [lambdaf]
  Vf/1 -> Sum/1, [vf]
  Va/1 -> Sum1/2, [va]
  [va] -> Product2/1
  [arm_ct] -> Product2/2
  Product2/1 -> Sum4/1
  [vf] -> Product3/1
  [field_ct] -> Product3/2
  Product3/1 -> Sum4/2
  Sum4/1 -> Pe/1
  [load_torque] -> Product4/1
  [speed] -> Product4/2
  Product4/1 -> Pm/1
  [arm_ct] -> Math Function1/1
  Math Function1/1 -> Gain8/1
  Gain8/1 -> Sum5/1
  [field_ct] -> Math Function2/1
  Math Function2/1 -> Gain9/1
  Gain9/1 -> Sum5/2
  Sum5/1 -> Plosses/1
  Integrator2/1 -> Speed/1, [speed], Integrator3/1
  Tload/1 -> [load_torque]

== system Boeing787_Yue/Hydraulic/Center Hydraulic System/DC Speed Servo1/DC Machine ==
  note: Armature Current ia
  note: Field Current If
  Vf : Inport
  Va : Inport  Port=2
  Tload : Inport  Port=3
  Gain : Gain  Gain=Rfsh
  Gain1 : Gain  Gain=1/Lfsh
  Gain2 : Gain  Gain=Ra
  Gain3 : Gain  Gain=1/La
  Gain4 : Gain  Gain=1/J
  Gain7 : Gain  Gain=Lmsh
  Gain8 : Gain  Gain=Ra
  Gain9 : Gain  Gain=Rfsh
  Integrator : Integrator
  Integrator1 : Integrator
  Integrator2 : Integrator  InitialCondition=1  LimitOutput=on  LowerSaturationLimit=1
  Integrator3 : Integrator  ZeroCross=off
  Math Function1 : Math  Operator=square  SaturateOnIntegerOverflow=on
  Math Function2 : Math  Operator=square  SaturateOnIntegerOverflow=on
  Product{,1..4} (5 alike) : Product  RndMeth=Zero
  Sum : Sum  Inputs=|+-
  Sum1 : Sum  Inputs=-+-
  Sum2 : Sum  Inputs=+-
  Sum4 : Sum  Inputs=|++
  Sum5 : Sum  Inputs=|++
  Terminator : Terminator
  If : Outport
  Ia : Outport  Port=2
  Pe : Outport  Port=3
  Pm : Outport  Port=4
  Plosses : Outport  Port=5
  Te : Outport  Port=6
  Speed : Outport  Port=7
  theta : Outport  Port=8
  wires:
  Integrator3/1 -> Terminator/1, theta/1
  Gain/1 -> Sum/2
  Sum/1 -> Gain1/1
  Integrator/1 -> Gain/1, [field_ct], If/1
  Sum1/1 -> Gain3/1
  Gain3/1 -> Integrator1/1
  Integrator1/1 -> Gain2/1, [arm_ct], Ia/1
  Product1/1 -> Sum2/1, Te/1
  Sum2/1 -> Gain4/1
  Gain4/1 -> Integrator2/1
  Gain1/1 -> Integrator/1
  Product/1 -> Sum1/1
  Gain2/1 -> Sum1/3
  [lambdaf] -> Product1/1
  [arm_ct] -> Product1/2
  [load_torque] -> Sum2/2
  [speed] -> Product/2
  [lambdaf] -> Product/1
  [field_ct] -> Gain7/1
  Gain7/1 -> [lambdaf]
  Vf/1 -> Sum/1, [vf]
  Va/1 -> Sum1/2, [va]
  [va] -> Product2/1
  [arm_ct] -> Product2/2
  Product2/1 -> Sum4/1
  [vf] -> Product3/1
  [field_ct] -> Product3/2
  Product3/1 -> Sum4/2
  Sum4/1 -> Pe/1
  [load_torque] -> Product4/1
  [speed] -> Product4/2
  Product4/1 -> Pm/1
  [arm_ct] -> Math Function1/1
  Math Function1/1 -> Gain8/1
  Gain8/1 -> Sum5/1
  [field_ct] -> Math Function2/1
  Math Function2/1 -> Gain9/1
  Gain9/1 -> Sum5/2
  Sum5/1 -> Plosses/1
  Integrator2/1 -> Speed/1, [speed], Integrator3/1
  Tload/1 -> [load_torque]

== system Boeing787_Yue/Hydraulic/Left Hydraulic System/DC Speed Servo/DC Machine ==
  note: Armature Current ia
  note: Field Current If
  Vf : Inport
  Va : Inport  Port=2
  Tload : Inport  Port=3
  Gain : Gain  Gain=Rfsh
  Gain1 : Gain  Gain=1/Lfsh
  Gain2 : Gain  Gain=Ra
  Gain3 : Gain  Gain=1/La
  Gain4 : Gain  Gain=1/J
  Gain7 : Gain  Gain=Lmsh
  Gain8 : Gain  Gain=Ra
  Gain9 : Gain  Gain=Rfsh
  Integrator : Integrator
  Integrator1 : Integrator
  Integrator2 : Integrator  InitialCondition=1  LimitOutput=on  LowerSaturationLimit=1
  Integrator3 : Integrator  ZeroCross=off
  Math Function1 : Math  Operator=square  SaturateOnIntegerOverflow=on
  Math Function2 : Math  Operator=square  SaturateOnIntegerOverflow=on
  Product{,1..4} (5 alike) : Product  RndMeth=Zero
  Scope : Scope
      settings: SaveName=ScopeData3
  Sum : Sum  Inputs=|+-
  Sum1 : Sum  Inputs=-+-
  Sum2 : Sum  Inputs=+-
  Sum4 : Sum  Inputs=|++
  Sum5 : Sum  Inputs=|++
  Terminator : Terminator
  If : Outport
  Ia : Outport  Port=2
  Pe : Outport  Port=3
  Pm : Outport  Port=4
  Plosses : Outport  Port=5
  Te : Outport  Port=6
  Speed : Outport  Port=7
  theta : Outport  Port=8
  wires:
  Integrator3/1 -> Terminator/1, theta/1
  Gain/1 -> Sum/2
  Sum/1 -> Gain1/1
  Integrator/1 -> Gain/1, [field_ct], If/1
  Sum1/1 -> Gain3/1
  Gain3/1 -> Integrator1/1
  Integrator1/1 -> Gain2/1, [arm_ct], Ia/1
  Product1/1 -> Scope/1, Sum2/1, Te/1
  Sum2/1 -> Gain4/1
  Gain4/1 -> Integrator2/1
  Gain1/1 -> Integrator/1
  Product/1 -> Sum1/1
  Gain2/1 -> Sum1/3
  [lambdaf] -> Product1/1
  [arm_ct] -> Product1/2
  [load_torque] -> Sum2/2
  [speed] -> Product/2
  [lambdaf] -> Product/1
  [field_ct] -> Gain7/1
  Gain7/1 -> [lambdaf]
  Vf/1 -> Sum/1, [vf]
  Va/1 -> Sum1/2, [va]
  [va] -> Product2/1
  [arm_ct] -> Product2/2
  Product2/1 -> Sum4/1
  [vf] -> Product3/1
  [field_ct] -> Product3/2
  Product3/1 -> Sum4/2
  Sum4/1 -> Pe/1
  [load_torque] -> Product4/1
  [speed] -> Product4/2
  Product4/1 -> Pm/1
  [arm_ct] -> Math Function1/1
  Math Function1/1 -> Gain8/1
  Gain8/1 -> Sum5/1
  [field_ct] -> Math Function2/1
  Math Function2/1 -> Gain9/1
  Gain9/1 -> Sum5/2
  Sum5/1 -> Plosses/1
  Integrator2/1 -> Speed/1, [speed], Integrator3/1
  Tload/1 -> [load_torque]

== system Boeing787_Yue/Hydraulic/Right Hydraulic System/DC Speed Servo/DC Machine ==
  note: Armature Current ia
  note: Field Current If
  Vf : Inport
  Va : Inport  Port=2
  Tload : Inport  Port=3
  Gain : Gain  Gain=Rfsh
  Gain1 : Gain  Gain=1/Lfsh
  Gain2 : Gain  Gain=Ra
  Gain3 : Gain  Gain=1/La
  Gain4 : Gain  Gain=1/J
  Gain7 : Gain  Gain=Lmsh
  Gain8 : Gain  Gain=Ra
  Gain9 : Gain  Gain=Rfsh
  Integrator : Integrator
  Integrator1 : Integrator
  Integrator2 : Integrator  InitialCondition=1  LimitOutput=on  LowerSaturationLimit=1
  Integrator3 : Integrator  ZeroCross=off
  Math Function1 : Math  Operator=square  SaturateOnIntegerOverflow=on
  Math Function2 : Math  Operator=square  SaturateOnIntegerOverflow=on
  Product{,1..4} (5 alike) : Product  RndMeth=Zero
  Sum : Sum  Inputs=|+-
  Sum1 : Sum  Inputs=-+-
  Sum2 : Sum  Inputs=+-
  Sum4 : Sum  Inputs=|++
  Sum5 : Sum  Inputs=|++
  Terminator : Terminator
  If : Outport
  Ia : Outport  Port=2
  Pe : Outport  Port=3
  Pm : Outport  Port=4
  Plosses : Outport  Port=5
  Te : Outport  Port=6
  Speed : Outport  Port=7
  theta : Outport  Port=8
  wires:
  Integrator3/1 -> Terminator/1, theta/1
  Gain/1 -> Sum/2
  Sum/1 -> Gain1/1
  Integrator/1 -> Gain/1, [field_ct], If/1
  Sum1/1 -> Gain3/1
  Gain3/1 -> Integrator1/1
  Integrator1/1 -> Gain2/1, [arm_ct], Ia/1
  Product1/1 -> Sum2/1, Te/1
  Sum2/1 -> Gain4/1
  Gain4/1 -> Integrator2/1
  Gain1/1 -> Integrator/1
  Product/1 -> Sum1/1
  Gain2/1 -> Sum1/3
  [lambdaf] -> Product1/1
  [arm_ct] -> Product1/2
  [speed] -> Product/2
  [lambdaf] -> Product/1
  [field_ct] -> Gain7/1
  Gain7/1 -> [lambdaf]
  Vf/1 -> Sum/1, [vf]
  Va/1 -> Sum1/2, [va]
  [va] -> Product2/1
  [arm_ct] -> Product2/2
  Product2/1 -> Sum4/1
  [vf] -> Product3/1
  [field_ct] -> Product3/2
  Product3/1 -> Sum4/2
  Sum4/1 -> Pe/1
  [load_torque] -> Product4/1
  [speed] -> Product4/2
  Product4/1 -> Pm/1
  [arm_ct] -> Math Function1/1
  Math Function1/1 -> Gain8/1
  Gain8/1 -> Sum5/1
  [field_ct] -> Math Function2/1
  Math Function2/1 -> Gain9/1
  Gain9/1 -> Sum5/2
  Sum5/1 -> Plosses/1
  Integrator2/1 -> Speed/1, [speed], Integrator3/1
  Tload/1 -> [load_torque]
  [load_torque] -> Sum2/2

== system Boeing787_Yue/ECS/Left Pack/Primary HX (air-air)/Air_properties_in_flows_hot_and_cold/air_properties_in_cold ==
  note: PLEASE NOTE that the air properties are based on the
      | inlet flow conditions rather than the average T and P.
      | Trying to base the properties on the average temperature
      | and even a constant pressure, the program did not work. One
      | suggestion is to average the inlet conditions with the outlet conditions
      | at a previous time step by using a memory block.x
  In_flow_bus_cold : Inport
  Bus Selector1 : BusSelector  OutputSignals=press_Pa,temp_C
  C to K : Bias  Bias=273
  Cp(P,T) : Lookup_n-D  BreakpointsForDimension1=AirProp.P  BreakpointsForDimension2=AirProp.T  BreakpointsForDimension3=[1]  Table=AirProp.Cp_pt  RndMeth=Simplest  InputSameDT=on
  Cp_pt_hot : Display
  Gain1 : Gain  Gain=1000
  Pa to kPa : Gain  Gain=10^-3
  Pr(P,T) : Lookup_n-D  BreakpointsForDimension1=AirProp.P  BreakpointsForDimension2=AirProp.T  BreakpointsForDimension3=[1]  Table=AirProp.Pr_pt  RndMeth=Simplest  InputSameDT=on
  Pr_pt_hot : Display
  Rho(P,T) : Lookup_n-D  BreakpointsForDimension1=AirProp.P  BreakpointsForDimension2=AirProp.T  BreakpointsForDimension3=[1]  Table=AirProp.Rho_pt  RndMeth=Simplest  InputSameDT=on
  Rho_pt_hot : Display
  k(P,T) : Lookup_n-D  BreakpointsForDimension1=AirProp.P  BreakpointsForDimension2=AirProp.T  BreakpointsForDimension3=[1]  Table=AirProp.k_pt  RndMeth=Simplest  InputSameDT=on
  k_pt_hot : Display
  mu(P,T) : Lookup_n-D  BreakpointsForDimension1=AirProp.P  BreakpointsForDimension2=AirProp.T  BreakpointsForDimension3=[1]  Table=AirProp.mu_pt  RndMeth=Simplest  InputSameDT=on
  mu_pt_hot : Display
  rho_air_kgm-3 : Outport
  cp_air_Jkg-1K-1 : Outport  Port=2
  mu_air_Pa.s : Outport  Port=3
  K_air_Wm-1K-2 : Outport  Port=4
  Pr : Outport  Port=5
  wires:
  In_flow_bus_cold/1 -> Bus Selector1/1
  C to K/1 -> Rho(P,T)/2, Pr(P,T)/2, k(P,T)/2, mu(P,T)/2, Cp(P,T)/2
  Bus Selector1/1 -> Pa to kPa/1  "<press_Pa>"
  Bus Selector1/2 -> C to K/1  "<temp_C>"
  Pa to kPa/1 -> Rho(P,T)/1, Cp(P,T)/1, mu(P,T)/1, Pr(P,T)/1, k(P,T)/1  "press_kPa"
  Rho(P,T)/1 -> Rho_pt_hot/1, rho_air_kgm-3/1
  Pr(P,T)/1 -> Pr_pt_hot/1, Pr/1
  k(P,T)/1 -> k_pt_hot/1, K_air_Wm-1K-2/1
  mu(P,T)/1 -> mu_pt_hot/1, mu_air_Pa.s/1
  Cp(P,T)/1 -> Cp_pt_hot/1, Gain1/1
  Gain1/1 -> cp_air_Jkg-1K-1/1

== system Boeing787_Yue/ECS/Left Pack/Primary HX (air-air)/Air_properties_in_flows_hot_and_cold/air_properties_in_hot ==
  note: PLEASE NOTE that the air properties are based on the
      | inlet flow conditions rather than the average T and P.
      | Trying to base the properties on the average temperature
      | and even a constant pressure, the program did not work. One
      | suggestion is to average the inlet conditions with the outlet conditions
      | at a previous time step by using a memory block.x
  In_flow_bus_hot : Inport
  Bus Selector : BusSelector  OutputSignals=pres_Pa,temp_C
  C to K : Bias  Bias=273
  Cp(P,T) : Lookup_n-D  BreakpointsForDimension1=AirProp.P  BreakpointsForDimension2=AirProp.T  BreakpointsForDimension3=[1]  Table=AirProp.Cp_pt  RndMeth=Simplest  InputSameDT=on
  Cp_pt_hot : Display
  Gain : Gain  Gain=1000
  Pa to kPa : Gain  Gain=10^-3
  Pr(P,T) : Lookup_n-D  BreakpointsForDimension1=AirProp.P  BreakpointsForDimension2=AirProp.T  BreakpointsForDimension3=[1]  Table=AirProp.Pr_pt  RndMeth=Simplest  InputSameDT=on
  Pr_pt_hot : Display
  Rho(P,T) : Lookup_n-D  BreakpointsForDimension1=AirProp.P  BreakpointsForDimension2=AirProp.T  BreakpointsForDimension3=[1]  Table=AirProp.Rho_pt  RndMeth=Simplest  InputSameDT=on
  Rho_pt_hot : Display
  k(P,T) : Lookup_n-D  BreakpointsForDimension1=AirProp.P  BreakpointsForDimension2=AirProp.T  BreakpointsForDimension3=[1]  Table=AirProp.k_pt  RndMeth=Simplest  InputSameDT=on
  k_pt_hot : Display
  mu(P,T) : Lookup_n-D  BreakpointsForDimension1=AirProp.P  BreakpointsForDimension2=AirProp.T  BreakpointsForDimension3=[1]  Table=AirProp.mu_pt  RndMeth=Simplest  InputSameDT=on
  mu_pt_hot : Display
  rho_air_kgm-3 : Outport
  cp_air_Jkg-1K-1 : Outport  Port=2
  mu_air_Pa.s : Outport  Port=3
  K_air_Wm-1K-2 : Outport  Port=4
  Pr : Outport  Port=5
  wires:
  In_flow_bus_hot/1 -> Bus Selector/1
  C to K/1 -> Rho(P,T)/2, Pr(P,T)/2, k(P,T)/2, mu(P,T)/2, Cp(P,T)/2
  Bus Selector/1 -> Pa to kPa/1  "<pres_Pa>"
  Bus Selector/2 -> C to K/1  "<temp_C>"
  Pa to kPa/1 -> Rho(P,T)/1, Cp(P,T)/1, mu(P,T)/1, Pr(P,T)/1, k(P,T)/1  "press_kPa"
  Rho(P,T)/1 -> Rho_pt_hot/1, rho_air_kgm-3/1
  Pr(P,T)/1 -> Pr/1, Pr_pt_hot/1
  k(P,T)/1 -> K_air_Wm-1K-2/1, k_pt_hot/1
  mu(P,T)/1 -> mu_air_Pa.s/1, mu_pt_hot/1
  Cp(P,T)/1 -> Gain/1, Cp_pt_hot/1
  Gain/1 -> cp_air_Jkg-1K-1/1

== system Boeing787_Yue/ECS/Left Pack/Primary HX (air-air)/HX_and_Fin_paramters/Fin_parameters ==
  Constant : Constant  Value=l_fin
  Constant1 : Constant  Value=t_fin
  Constant2 : Constant  Value=s_fin
  Constant3 : Constant  Value=h_fin
  Constant4 : Constant  Value=K_n
  Constant5 : Constant  Value=eta_f
  Fin_length_m : Outport
  Fin_thickness_m : Outport  Port=2
  Fin_free_flow_width_m : Outport  Port=3
  Fin_free_flow_height_m : Outport  Port=4
  K_fin_Wm-1K-1 : Outport  Port=5
  Fin_eff : Outport  Port=6
  wires:
  Constant1/1 -> Fin_thickness_m/1
  Constant2/1 -> Fin_free_flow_width_m/1
  Constant3/1 -> Fin_free_flow_height_m/1
  Constant4/1 -> K_fin_Wm-1K-1/1
  Constant5/1 -> Fin_eff/1
  Constant/1 -> Fin_length_m/1

== system Boeing787_Yue/ECS/Left Pack/Primary HX (air-air)/HX_and_Fin_paramters/HX_parameters ==
  Other_HX_parameters : Inport
  Fin_parameters : Inport  Port=2
  Bus Selector : BusSelector  OutputSignals=L_hx
  Calculating the no of passages per fluid flow : Subsystem
  Calculating the total number of fins per HX per fluid flow : Subsystem
  Calculating total free flow area per flow : Subsystem
  Constant3 : Constant  Value=K_p
  Constant4 : Constant  Value=cp_hx
  Constant5 : Constant  Value=m_cm
  Display : Display
  Display1 : Display
  Display2 : Display
  tot_free_flow_area_m^2 : Outport
  tot_length_in_direc_of_flow_m : Outport  Port=2
  tot_no_of_fins_per_HX_per_flow : Outport  Port=3
  K_hx_Wm-1K-1 : Outport  Port=4
  cp_hx_Jkg-1K-1 : Outport  Port=5
  m_hx_kg : Outport  Port=6
  wires:
  Bus Selector/1 -> tot_length_in_direc_of_flow_m/1  "<L_hx>"
  Calculating the total number of fins per HX per fluid flow/1(Tot_no_of_fins_per_HX_per_flow) -> Display2/1, tot_no_of_fins_per_HX_per_flow/1  "N_f"
  Calculating total free flow area per flow/1(Total_free_flow_area) -> Display/1, tot_free_flow_area_m^2/1  "A"
  Calculating the no of passages per fluid flow/1(N_passages_per_flow) -> Display1/1, Calculating the total number of fins per HX per fluid flow/3(N_passages_per_flow), Calculating total free flow area per flow/3(N_passages_per_flow)
  Fin_parameters/1 -> Calculating the total number of fins per HX per fluid flow/2(Fin_parameters), Calculating total free flow area per flow/2(Fin_parameters), Calculating the no of passages per fluid flow/2(Fin_parameters)
  Other_HX_parameters/1 -> Bus Selector/1, Calculating the total number of fins per HX per fluid flow/1(Raw_HX_parameters), Calculating total free flow area per flow/1(Raw_HX_parameters), Calculating the no of passages per fluid flow/1(Raw_HX_parameters)
  Constant5/1 -> m_hx_kg/1
  Constant3/1 -> K_hx_Wm-1K-1/1
  Constant4/1 -> cp_hx_Jkg-1K-1/1

== system Boeing787_Yue/ECS/Left Pack/Primary HX (air-air)/HX_and_Fin_paramters/Other_HX_parameters2 ==
  Bus Creator : BusCreator
  Length in flow direction : Constant  Value=L_hx
  plate thickness : Constant  Value=t_p
  total height : Constant  Value=H_hx
  width : Constant  Value=W_hx
  Out1 : Outport
  wires:
  Bus Creator/1 -> Out1/1
  plate thickness/1 -> Bus Creator/4  "t_p"
  total height/1 -> Bus Creator/3  "H_hx"
  width/1 -> Bus Creator/2  "W_hx"
  Length in flow direction/1 -> Bus Creator/1  "L_hx"

== system Boeing787_Yue/ECS/Left Pack/Secondary HX (air-air)1/Air_properties_in_flows_hot_and_cold/air_properties_in_cold ==
  note: PLEASE NOTE that the air properties are based on the
      | inlet flow conditions rather than the average T and P.
      | Trying to base the properties on the average temperature
      | and even a constant pressure, the program did not work. One
      | suggestion is to average the inlet conditions with the outlet conditions
      | at a previous time step by using a memory block.x
  In_flow_bus_cold : Inport
  Bus Selector1 : BusSelector  OutputSignals=press_Pa,temp_C
  C to K : Bias  Bias=273
  Cp(P,T) : Lookup_n-D  BreakpointsForDimension1=AirProp.P  BreakpointsForDimension2=AirProp.T  BreakpointsForDimension3=[1]  Table=AirProp.Cp_pt  RndMeth=Simplest  InputSameDT=on
  Cp_pt_hot : Display
  Gain1 : Gain  Gain=1000
  Pa to kPa : Gain  Gain=10^-3
  Pr(P,T) : Lookup_n-D  BreakpointsForDimension1=AirProp.P  BreakpointsForDimension2=AirProp.T  BreakpointsForDimension3=[1]  Table=AirProp.Pr_pt  RndMeth=Simplest  InputSameDT=on
  Pr_pt_hot : Display
  Rho(P,T) : Lookup_n-D  BreakpointsForDimension1=AirProp.P  BreakpointsForDimension2=AirProp.T  BreakpointsForDimension3=[1]  Table=AirProp.Rho_pt  RndMeth=Simplest  InputSameDT=on
  Rho_pt_hot : Display
  k(P,T) : Lookup_n-D  BreakpointsForDimension1=AirProp.P  BreakpointsForDimension2=AirProp.T  BreakpointsForDimension3=[1]  Table=AirProp.k_pt  RndMeth=Simplest  InputSameDT=on
  k_pt_hot : Display
  mu(P,T) : Lookup_n-D  BreakpointsForDimension1=AirProp.P  BreakpointsForDimension2=AirProp.T  BreakpointsForDimension3=[1]  Table=AirProp.mu_pt  RndMeth=Simplest  InputSameDT=on
  mu_pt_hot : Display
  rho_air_kgm-3 : Outport
  cp_air_Jkg-1K-1 : Outport  Port=2
  mu_air_Pa.s : Outport  Port=3
  K_air_Wm-1K-2 : Outport  Port=4
  Pr : Outport  Port=5
  wires:
  In_flow_bus_cold/1 -> Bus Selector1/1
  C to K/1 -> Rho(P,T)/2, Pr(P,T)/2, k(P,T)/2, mu(P,T)/2, Cp(P,T)/2
  Bus Selector1/1 -> Pa to kPa/1  "<press_Pa>"
  Bus Selector1/2 -> C to K/1  "<temp_C>"
  Pa to kPa/1 -> Rho(P,T)/1, Cp(P,T)/1, mu(P,T)/1, Pr(P,T)/1, k(P,T)/1  "press_kPa"
  Rho(P,T)/1 -> Rho_pt_hot/1, rho_air_kgm-3/1
  Pr(P,T)/1 -> Pr_pt_hot/1, Pr/1
  k(P,T)/1 -> k_pt_hot/1, K_air_Wm-1K-2/1
  mu(P,T)/1 -> mu_pt_hot/1, mu_air_Pa.s/1
  Cp(P,T)/1 -> Cp_pt_hot/1, Gain1/1
  Gain1/1 -> cp_air_Jkg-1K-1/1

== system Boeing787_Yue/ECS/Left Pack/Secondary HX (air-air)1/Air_properties_in_flows_hot_and_cold/air_properties_in_hot ==
  note: PLEASE NOTE that the air properties are based on the
      | inlet flow conditions rather than the average T and P.
      | Trying to base the properties on the average temperature
      | and even a constant pressure, the program did not work. One
      | suggestion is to average the inlet conditions with the outlet conditions
      | at a previous time step by using a memory block.x
  In_flow_bus_hot : Inport
  Bus Selector : BusSelector  OutputSignals=pres_Pa,temp_C
  C to K : Bias  Bias=273
  Cp(P,T) : Lookup_n-D  BreakpointsForDimension1=AirProp.P  BreakpointsForDimension2=AirProp.T  BreakpointsForDimension3=[1]  Table=AirProp.Cp_pt  RndMeth=Simplest  InputSameDT=on
  Cp_pt_hot : Display
  Gain : Gain  Gain=1000
  Pa to kPa : Gain  Gain=10^-3
  Pr(P,T) : Lookup_n-D  BreakpointsForDimension1=AirProp.P  BreakpointsForDimension2=AirProp.T  BreakpointsForDimension3=[1]  Table=AirProp.Pr_pt  RndMeth=Simplest  InputSameDT=on
  Pr_pt_hot : Display
  Rho(P,T) : Lookup_n-D  BreakpointsForDimension1=AirProp.P  BreakpointsForDimension2=AirProp.T  BreakpointsForDimension3=[1]  Table=AirProp.Rho_pt  RndMeth=Simplest  InputSameDT=on
  Rho_pt_hot : Display
  k(P,T) : Lookup_n-D  BreakpointsForDimension1=AirProp.P  BreakpointsForDimension2=AirProp.T  BreakpointsForDimension3=[1]  Table=AirProp.k_pt  RndMeth=Simplest  InputSameDT=on
  k_pt_hot : Display
  mu(P,T) : Lookup_n-D  BreakpointsForDimension1=AirProp.P  BreakpointsForDimension2=AirProp.T  BreakpointsForDimension3=[1]  Table=AirProp.mu_pt  RndMeth=Simplest  InputSameDT=on
  mu_pt_hot : Display
  rho_air_kgm-3 : Outport
  cp_air_Jkg-1K-1 : Outport  Port=2
  mu_air_Pa.s : Outport  Port=3
  K_air_Wm-1K-2 : Outport  Port=4
  Pr : Outport  Port=5
  wires:
  In_flow_bus_hot/1 -> Bus Selector/1
  C to K/1 -> Rho(P,T)/2, Pr(P,T)/2, k(P,T)/2, mu(P,T)/2, Cp(P,T)/2
  Bus Selector/1 -> Pa to kPa/1  "<pres_Pa>"
  Bus Selector/2 -> C to K/1  "<temp_C>"
  Pa to kPa/1 -> Rho(P,T)/1, Cp(P,T)/1, mu(P,T)/1, Pr(P,T)/1, k(P,T)/1  "press_kPa"
  Rho(P,T)/1 -> Rho_pt_hot/1, rho_air_kgm-3/1
  Pr(P,T)/1 -> Pr/1, Pr_pt_hot/1
  k(P,T)/1 -> K_air_Wm-1K-2/1, k_pt_hot/1
  mu(P,T)/1 -> mu_air_Pa.s/1, mu_pt_hot/1
  Cp(P,T)/1 -> Gain/1, Cp_pt_hot/1
  Gain/1 -> cp_air_Jkg-1K-1/1

== system Boeing787_Yue/ECS/Left Pack/Secondary HX (air-air)1/HX_and_Fin_paramters/Fin_parameters ==
  Constant : Constant  Value=l_fin
  Constant1 : Constant  Value=t_fin
  Constant2 : Constant  Value=s_fin
  Constant3 : Constant  Value=h_fin
  Constant4 : Constant  Value=K_n
  Constant5 : Constant  Value=eta_f
  Fin_length_m : Outport
  Fin_thickness_m : Outport  Port=2
  Fin_free_flow_width_m : Outport  Port=3
  Fin_free_flow_height_m : Outport  Port=4
  K_fin_Wm-1K-1 : Outport  Port=5
  Fin_eff : Outport  Port=6
  wires:
  Constant1/1 -> Fin_thickness_m/1
  Constant2/1 -> Fin_free_flow_width_m/1
  Constant3/1 -> Fin_free_flow_height_m/1
  Constant4/1 -> K_fin_Wm-1K-1/1
  Constant5/1 -> Fin_eff/1
  Constant/1 -> Fin_length_m/1
